simulink model "ModeloOpal"  (R2017a)
settings: Solver=ode4  StartTime=0.0  StopTime=inf  FixedStep=Ts  RelTol=1e-3  EnableMultiTasking=on
PostLoadFcn:
  | Ts=1/100080;L=1.8e-3;w=2*pi*60;C=20e-6;
  | 
  | load('CycleFTP75.mat')
  | 
  | Vel=Cycle(:,1);
  | Acc=Cycle(:,2);
InitFcn:
  | Ts=1/100080;L=1.8e-3;w=2*pi*60;C=20e-6;
  | 
  | load('CycleFTP75.mat')
  | 
  | Vel=Cycle(:,1);
  | Acc=Cycle(:,2);
undefined symbols (not defined in the file): DiscIntNeverNeededParam, OP4510_1B_Ch00, OP4510_2A_Ch00, OP4510_2A_Ch08, OP4510_2B_Ch00, OP4510_2B_Ch08, sizecont
libraries: rtlab x29, simulink x5, dspswit3 x2
(part 1 of 2)
Description:
  | Model of a simple control system for use iin training.
settings Model: Creator=Paul Baracos  LastModifiedBy=LIFAE
settings SolverCC: InsertRTBMode=Never (minimum delay)
settings DataIOCC: LimitDataPoints=on  SaveFormat=Array  SaveOutput=off  SaveTime=off  SignalLoggingName=sigsOut
settings OptimizationCC: BlockReduction=off  BooleanDataType=off  OptimizeBlockIOStorage=off  BufferReuse=off  GlobalBufferReuse=off  ExpressionFolding=off  LocalBlockOutputs=off  InitFltsAndDblsToZero=on  LifeSpan=inf
settings DebuggingCC: SaveWithParameterizedLinksMsg=none  UnderspecifiedInitializationDetection=Classic  MergeDetectMultiDrivingBlocksExec=none  SignalResolutionControl=TryResolveAllWithWarning  MultiTaskDSMMsg=warning  MultiTaskCondExecSysMsg=none  FcnCallInpInsideContextMsg=warning  SFUnexpectedBacktrackingDiag=warning  SFNoUnconditionalDefaultTransitionDiag=warning  SFExecutionAtInitializationDiag=none
settings HardwareCC: ProdBitPerPointer=32  ProdBitPerSizeT=32  ProdBitPerPtrDiffT=32  ProdLargestAtomicFloat=None  ProdIntDivRoundTo=Undefined  ProdEndianess=Unspecified  ProdWordSize=32  ProdHWDeviceType=32-bit Generic  TargetBitPerPointer=64  TargetBitPerSizeT=64  TargetBitPerPtrDiffT=64  TargetLongLongMode=on  TargetIntDivRoundTo=Zero  TargetEndianess=LittleEndian  TargetWordSize=64  TargetHWDeviceType=MATLAB Host  ProdEqTarget=off
settings ModelReferenceCC: PropagateSignalLabelsOutOfModel=off
settings GRTTargetCC: TargetFcnLib=ansi_tfl_tmw.mat  TargetLangStandard=C89/C90 (ANSI)  CombineOutputUpdateFcns=off  GRTInterface=on
settings ConfigComp: CovMetricSettings=dw  CovSaveCumulativeToWorkspaceVar=on  CovSaveSingleToWorkspaceVar=on  CovExternalEMLEnable=off

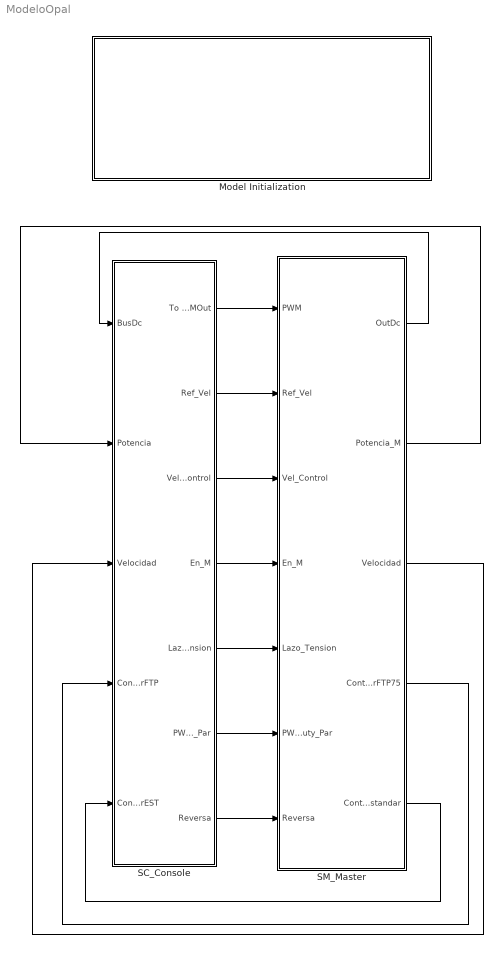
== system ModeloOpal ==
  Model Initialization : Subsystem  AncestorBlock=artemis/Tools /Misc/Model Initialization  mask(Model Functions){InitFcnX=|, prel=off, posl=on, inif=on, strf=off}
      mask InitFcnX=|
      | Ts=1/100080;L=1.8e-3;w=2*pi*60;C=20e-6;
      |
      | load('CycleFTP75.mat')
      |
      | Vel=Cycle(:,1);
      | Acc=Cycle(:,2);
      mask prompts: InitFcnX "Initialisation"; prel "Preload Function"; posl "PostLoad Function"; inif "InitFcn"; strf "StartFcn"
      mask init:
      | currentBlock = gcb;
      | root = bdroot(currentBlock);
      | 
      | if ~strcmp(get_param(root,'BlockDiagramType'),'library')
      |     if prel==1
      |         set_param(root, 'PreLoadFcn', InitFcnX);
      |     else
      |         set_param(root, 'PreLoadFcn', '');
      |     end
      |     if inif==1
      |         set_param(root, 'InitFcn', InitFcnX);
      |     else
      |         set_param(root, 'InitFcn', '');
      |     end
      |     if strf==1
      |         set_param(root, 'StartFcn', InitFcnX);
      |     else
      |         set_param(root, 'StartFcn', '');
      |     end
      |     if posl==1
      |         set_param(root, 'PostLoadFcn', InitFcnX);
      |     else
      |         set_param(root, 'PostLoadFcn', '');
      |     end
      | end
      | 
      | pos = get_param(currentBlock, 'Position');
      | width = pos(3) - pos(1); height = pos(4) - pos(2);
      | txt = [ upper(root) '\n' '- InitFcn. . . . . '  get_param(root, 'InitFcn') ];
      settings: CopyFcn=set_param(gcb,'LinkStatus','inactive')
      mask Display: text(5, height*0.5, txt, 'horizontalAlignment', 'left', 'verticalAlignment', 'middle') ;
  SC_Console : Subsystem
  SM_Master : Subsystem
  wires:
  SM_Master/1("OutDc ") -> SC_Console/1(BusDc)
  SM_Master/2(Potencia_M) -> SC_Console/2(Potencia)
  SC_Console/1(To PWMOut) -> SM_Master/1("PWM ")
  SM_Master/3(Velocidad) -> SC_Console/3(Velocidad)
  SM_Master/4(ContadorFTP75) -> SC_Console/4(ContadorFTP)
  SM_Master/5(ContadorEstandar) -> SC_Console/5(ContadorEST)
  SC_Console/2(Ref_Vel) -> SM_Master/2(Ref_Vel)
  SC_Console/3(Vel_Control) -> SM_Master/3(Vel_Control)
  SC_Console/4(En_M) -> SM_Master/4(En_M)
  SC_Console/5("Lazo_Tension ") -> SM_Master/5(Lazo_Tension)
  SC_Console/6(PWM_Duty_Par) -> SM_Master/6(PWM_Duty_Par)
  SC_Console/7(Reversa) -> SM_Master/7(Reversa)

== system ModeloOpal/Model Initialization ==

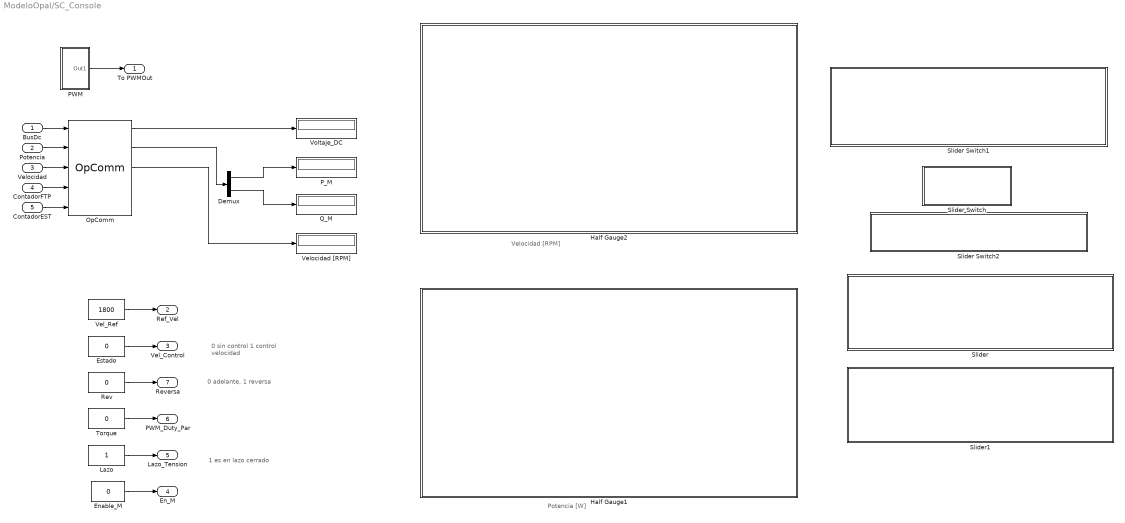
== system ModeloOpal/SC_Console ==
  note: Velocidad [RPM]
  note: 0 sin control
      | 1 control velocidad
  note: 0 adelante, 1 reversa
  note: 1 es en lazo cerrado
  note: Potencia [W]
  BusDc : Inport
  Potencia : Inport  Port=2
  Velocidad : Inport  Port=3
  ContadorFTP : Inport  Port=4
  ContadorEST : Inport  Port=5
  Demux : Demux  Outputs=2
  Enable_M : Constant  Value=0
  Estado : Constant  Value=0
  Half Gauge1 : Subsystem  DialogController=hmiCreateDDGDialog  IsWebBlock=on  mask(MWDashboardBlock){webBlockId=9bf2f812-ab57-4af6-888e-ff456dd2f0e9, webBlockType=semicirculargauge, ShowInLibBrowser=on, ShowInitialText=on, HMISrcModelName=EV}
      mask prompts: webBlockId "WebBlock Id"; webBlockType "WebBlock Type"; HMISrcModelName "Source Model"
      mask help: SimulinkHMI:dialogs:SemicircularGaugeDialogDesc
      mask Help: helpview([docroot '/mapfiles/simulink.map'], 'hmi_half_gauge')
      mask Display:
      | if strcmp(get_param(bdroot(gcb),'BlockDiagramType'), 'library')
      |     image([(matlabroot) '/toolbox/simulink/hmi/icons/SemicircularGauge.png']);
      | end
  Half Gauge2 : Subsystem  DialogController=hmiCreateDDGDialog  IsWebBlock=on  mask(MWDashboardBlock){webBlockId=4c0e6855-45c1-4807-b490-75edbe862d8f, webBlockType=semicirculargauge, ShowInLibBrowser=on, ShowInitialText=on, HMISrcModelName=EV}
      mask prompts: webBlockId "WebBlock Id"; webBlockType "WebBlock Type"; HMISrcModelName "Source Model"
      mask help: SimulinkHMI:dialogs:SemicircularGaugeDialogDesc
      mask Help: helpview([docroot '/mapfiles/simulink.map'], 'hmi_half_gauge')
      mask Display:
      | if strcmp(get_param(bdroot(gcb),'BlockDiagramType'), 'library')
      |     image([(matlabroot) '/toolbox/simulink/hmi/icons/SemicircularGauge.png']);
      | end
  Lazo : Constant
  OpComm : rtlab/OpComm  nbport=5  groupe_acq=1  subsys_rate=0  st=0  Synchronization=on  Interpolation=on  Threshold=1.0  Missed_Data=off  Sim_Time=off  Samples=off  dynSigOut=off  from_console=0  warning_done=off  writeOpCommFile=off  Offset=off
      settings: SourceProductName=RT-LAB
  PWM : Subsystem
  P_M : Display
  Q_M : Display
  Rev : Constant  Value=0
  Slider : Subsystem  DialogController=hmiCreateDDGDialog  IsWebBlock=on  mask(MWDashboardBlock){webBlockId=662892dd-7b3a-463b-8f2b-6a3bb7b3c375, webBlockType=slider, ShowInLibBrowser=on, ShowInitialText=on, HMISrcModelName=EV}
      mask prompts: webBlockId "WebBlock Id"; webBlockType "WebBlock Type"; HMISrcModelName "Source Model"
      mask help: SimulinkHMI:dialogs:SliderDialogDesc
      mask Help: helpview([docroot '/mapfiles/simulink.map'], 'hmi_slider')
      mask Display:
      | if strcmp(get_param(bdroot(gcb),'BlockDiagramType'), 'library')
      |     image([(matlabroot) '/toolbox/simulink/hmi/icons/Slider.png']);
      | end
  Slider Switch : Subsystem  DialogController=hmiCreateDDGDialog  IsWebBlock=on  mask(MWDashboardBlock){webBlockId=e4e01401-8b8e-4eb0-8cfa-0b1290c49f07, webBlockType=sliderswitch, ShowInLibBrowser=on, ShowInitialText=on, HMISrcModelName=EV}
      mask prompts: webBlockId "WebBlock Id"; webBlockType "WebBlock Type"; HMISrcModelName "Source Model"
      mask help: SimulinkHMI:dialogs:SwitchDialogDesc
      mask Help: helpview([docroot '/mapfiles/simulink.map'], 'hmi_slider_switch')
      mask Display:
      | if strcmp(get_param(bdroot(gcb),'BlockDiagramType'), 'library')
      |     image([(matlabroot) '/toolbox/simulink/hmi/icons/SliderSwitch.png']);
      | end
  Slider Switch1 : Subsystem  DialogController=hmiCreateDDGDialog  IsWebBlock=on  mask(MWDashboardBlock){webBlockId=fdde9750-0d4e-4e96-acc9-80e84340a54d, webBlockType=sliderswitch, ShowInLibBrowser=on, ShowInitialText=on, HMISrcModelName=EV}
      mask prompts: webBlockId "WebBlock Id"; webBlockType "WebBlock Type"; HMISrcModelName "Source Model"
      mask help: SimulinkHMI:dialogs:SwitchDialogDesc
      mask Help: helpview([docroot '/mapfiles/simulink.map'], 'hmi_slider_switch')
      mask Display:
      | if strcmp(get_param(bdroot(gcb),'BlockDiagramType'), 'library')
      |     image([(matlabroot) '/toolbox/simulink/hmi/icons/SliderSwitch.png']);
      | end
  Slider Switch2 : Subsystem  DialogController=hmiCreateDDGDialog  IsWebBlock=on  mask(MWDashboardBlock){webBlockId=cc9abc73-cb6f-40c5-b477-d0f2468ee603, webBlockType=sliderswitch, ShowInLibBrowser=on, ShowInitialText=on, HMISrcModelName=EV}
      mask prompts: webBlockId "WebBlock Id"; webBlockType "WebBlock Type"; HMISrcModelName "Source Model"
      mask help: SimulinkHMI:dialogs:SwitchDialogDesc
      mask Help: helpview([docroot '/mapfiles/simulink.map'], 'hmi_slider_switch')
      mask Display:
      | if strcmp(get_param(bdroot(gcb),'BlockDiagramType'), 'library')
      |     image([(matlabroot) '/toolbox/simulink/hmi/icons/SliderSwitch.png']);
      | end
  Slider1 : Subsystem  DialogController=hmiCreateDDGDialog  IsWebBlock=on  mask(MWDashboardBlock){webBlockId=d9866bfa-8e08-4068-9fd6-1c09dd8bbfc2, webBlockType=slider, ShowInLibBrowser=on, ShowInitialText=on, HMISrcModelName=EV}
      mask prompts: webBlockId "WebBlock Id"; webBlockType "WebBlock Type"; HMISrcModelName "Source Model"
      mask help: SimulinkHMI:dialogs:SliderDialogDesc
      mask Help: helpview([docroot '/mapfiles/simulink.map'], 'hmi_slider')
      mask Display:
      | if strcmp(get_param(bdroot(gcb),'BlockDiagramType'), 'library')
      |     image([(matlabroot) '/toolbox/simulink/hmi/icons/Slider.png']);
      | end
  Torque : Constant  Value=0
  Vel_Ref : Constant  Value=1800
  Velocidad [RPM] : Display
  Voltaje_DC : Display
  To PWMOut : Outport
  Ref_Vel : Outport  Port=2
  Vel_Control : Outport  Port=3
  En_M : Outport  Port=4
  "Lazo_Tension " : Outport  Port=5
  PWM_Duty_Par : Outport  Port=6
  Reversa : Outport  Port=7
  wires:
  BusDc/1 -> OpComm/1
  OpComm/1 -> Voltaje_DC/1
  Potencia/1 -> OpComm/2
  OpComm/2 -> Demux/1
  Demux/1 -> P_M/1
  Demux/2 -> Q_M/1
  PWM/1(Out1) -> To PWMOut/1
  Enable_M/1 -> En_M/1
  Lazo/1 -> "Lazo_Tension "/1
  Torque/1 -> PWM_Duty_Par/1
  Velocidad/1 -> OpComm/3
  OpComm/3 -> Velocidad [RPM]/1
  ContadorFTP/1 -> OpComm/4
  Rev/1 -> Reversa/1
  Estado/1 -> Vel_Control/1
  Vel_Ref/1 -> Ref_Vel/1
  ContadorEST/1 -> OpComm/5

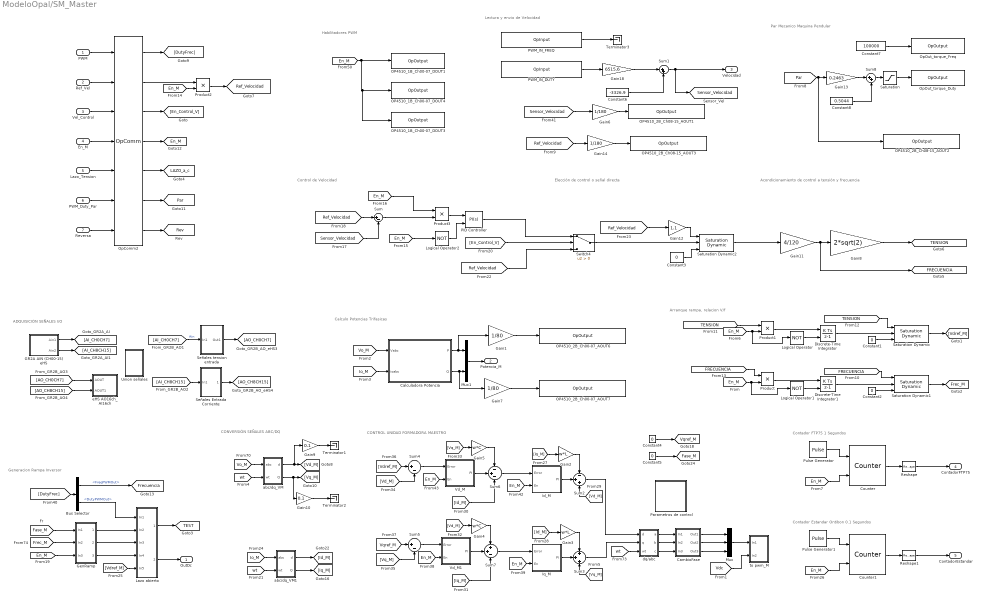
== system ModeloOpal/SM_Master ==
  note: Lectura y envio de Velocidad
  note: Calculo Potencias Trifasicas
  note: Generacion Rampa Inversor
  note: Arranque rampa, relacion V/f
  note: Par Mecanico Maquina Pendular
  note: Contador FTP75 1 Segundos
  note: Acondicionamiento de control a tensión y frecuencia
  note: Elección de control o señal directa
  note: Control de Velocidad
  note: Habilitadores PWM
  note: ADQUISICIÓN SEÑALES I/O
  note: CONVERSIÓN SEÑALES ABC/DQ
  note: CONTROL UNIDAD FORMADORA MAESTRO
  note: Contador Estandar Ontibon 0.1 Segundos
  "PWM " : Inport
  Ref_Vel : Inport  Port=2
  Vel_Control : Inport  Port=3
  En_M : Inport  Port=4
  Lazo_Tension : Inport  Port=5
  PWM_Duty_Par : Inport  Port=6
  Reversa : Inport  Port=7
  Bus Selector : BusSelector  OutputSignals=FreqPWMOut,DutyPWMOut
  Calculadora Potencia : Subsystem
  CambioFase : Subsystem
  Constant{1..5} (5 alike) : Constant  Value=0
  Constant6 : Constant  Value=-3326.9
  Constant7 : Constant  Value=100000
  Constant8 : Constant  Value=0.5044
  Counter : dspswit3/Counter  Direction=Up  CountEvent=Rising edge  CounterSize=User defined  MaxCount=2474  InitialCount=0  Output=Count  HitValue=sizecont-1  ResetInput=on  SamplesPerFrame=1  Ts=1  CntDtype=double  HitDtype=Logical
  Counter1 : dspswit3/Counter  Direction=Up  CountEvent=Rising edge  CounterSize=User defined  MaxCount=2474  InitialCount=0  Output=Count  HitValue=sizecont-1  ResetInput=on  SamplesPerFrame=1  Ts=1  CntDtype=double  HitDtype=Logical
  Discrete-Time Integrator : DiscreteIntegrator  ExternalReset=level  InitialConditionSetting=State (most efficient)  SampleTime=-1  ICPrevOutput=DiscIntNeverNeededParam  ICPrevScaledInput=DiscIntNeverNeededParam
  Discrete-Time Integrator1 : DiscreteIntegrator  ExternalReset=level  InitialConditionSetting=State (most efficient)  SampleTime=-1  ICPrevOutput=DiscIntNeverNeededParam  ICPrevScaledInput=DiscIntNeverNeededParam
  GR2A AIN (CH00-15) eHS : Subsystem
  Gain1 : Gain  Gain=1/80
  Gain10 : Gain  Gain=0.1
  Gain11 : Gain  Gain=4/120
  Gain12 : Gain  Gain=1.1
  Gain13 : Gain  Gain=0.2463
  Gain14 : Gain  Gain=1/180
  Gain18 : Gain  Gain=6515.6
  Gain2 : Gain  Gain=w*L
  Gain3 : Gain  Gain=w*L
  Gain4 : Gain  Gain=w*C
  Gain5 : Gain  Gain=w*C
  Gain6 : Gain  Gain=1/180
  Gain7 : Gain  Gain=1/80
  Gain8 : Gain  Gain=2*sqrt(2)  SaturateOnIntegerOverflow=on  OutDataTypeStr=Inherit: Same as input  ParamDataTypeStr=Inherit: Same as input
  Gain9 : Gain  Gain=0.1
  GenRamp : Subsystem
  Id_M : Subsystem
  Iq_M : Subsystem
  "Lazo abierto " : Subsystem
  Logical Operator : Logic  Operator=NOT  AllPortsSameDT=off  OutDataTypeStr=boolean
  Logical Operator1 : Logic  Operator=NOT  AllPortsSameDT=off  OutDataTypeStr=boolean
  Logical Operator2 : Logic  Operator=NOT  AllPortsSameDT=off  OutDataTypeStr=boolean
  Mux : Mux  Inputs=3
  Mux1 : Mux  Inputs=2
  OP4510_1B_Ch00-07_DOUT1 : rtlab/OpOutput  identifier_use=[]  identifier_hide=OP4510_1B_Ch00-07_DOUT1  nb_parents_identifier=0
      settings: SourceProductName=RT-LAB
  OP4510_1B_Ch00-07_DOUT3 : rtlab/OpOutput  identifier_use=[]  identifier_hide=OP4510_1B_Ch00-07_DOUT3  nb_parents_identifier=0
      settings: SourceProductName=RT-LAB
  OP4510_1B_Ch00-07_DOUT4 : rtlab/OpOutput  identifier_use=[]  identifier_hide=OP4510_1B_Ch00-07_DOUT4  nb_parents_identifier=0
      settings: SourceProductName=RT-LAB
  OP4510_2B_Ch00-07_AOUT6 : rtlab/OpOutput  identifier_use=[]  identifier_hide=OP4510_2B_Ch00-07_AOUT6  nb_parents_identifier=0
      settings: SourceProductName=RT-LAB
  OP4510_2B_Ch00-07_AOUT7 : rtlab/OpOutput  identifier_use=[]  identifier_hide=OP4510_2B_Ch00-07_AOUT7  nb_parents_identifier=0
      settings: SourceProductName=RT-LAB
  OP4510_2B_Ch08-15_AOUT1 : rtlab/OpOutput  identifier_use=[]  identifier_hide=OP4510_2B_Ch08-15_AOUT1  nb_parents_identifier=0
      settings: SourceProductName=RT-LAB
  OP4510_2B_Ch08-15_AOUT2 : rtlab/OpOutput  identifier_use=[]  identifier_hide=OP4510_2B_Ch08-15_AOUT2  nb_parents_identifier=0
      settings: SourceProductName=RT-LAB
  OP4510_2B_Ch08-15_AOUT3 : rtlab/OpOutput  identifier_use=[]  identifier_hide=OP4510_2B_Ch08-15_AOUT3  nb_parents_identifier=0
      settings: SourceProductName=RT-LAB
  OpComm2 : rtlab/OpComm  nbport=7  groupe_acq=1  subsys_rate=0  st=0  Synchronization=on  Interpolation=on  Threshold=1.0  Missed_Data=off  Sim_Time=off  Samples=off  dynSigOut=off  from_console=1  warning_done=off  writeOpCommFile=off  Offset=off
      settings: SourceProductName=RT-LAB
  OpOut_torque_Duty : rtlab/OpOutput  identifier_use=[]  identifier_hide=OpOut_torque_Duty  nb_parents_identifier=0
      settings: SourceProductName=RT-LAB
  OpOut_torque_Freq : rtlab/OpOutput  identifier_use=[]  identifier_hide=OpOut_torque_Freq  nb_parents_identifier=0
      settings: SourceProductName=RT-LAB
  PID Controller : simulink/Continuous/PID Controller  Controller=PI  TimeDomain=Continuous-time  SampleTime=-1  IntegratorMethod=Forward Euler  FilterMethod=Forward Euler  Form=Parallel  UseFilter=on  ControllerParametersSource=internal  P=0.502  I=21.7  D=0  N=100  InitialConditionSource=internal  InitialConditionForIntegrator=0  InitialConditionForFilter=0  ExternalReset=level  LimitOutput=off  UpperSaturationLimit=inf  LowerSaturationLimit=-inf  LinearizeAsGain=on  AntiWindupMode=none  Kb=1  TrackingMode=off  Kt=1  PParamMin=[]  PParamMax=[]  IParamMin=[]  IParamMax=[]  DParamMin=[]  DParamMax=[]  NParamMin=[]  NParamMax=[]  KbParamMin=[]  KbParamMax=[]  KtParamMin=[]  KtParamMax=[]  POutMin=[]  POutMax=[]  IOutMin=[]  IOutMax=[]  DOutMin=[]  DOutMax=[]  NOutMin=[]  NOutMax=[]  KbOutMin=[]  KbOutMax=[]  KtOutMin=[]  KtOutMax=[]  IntegratorOutMin=[]  IntegratorOutMax=[]  FilterOutMin=[]  FilterOutMax=[]  SumOutMin=[]  SumOutMax=[]  SumI1OutMin=[]  SumI1OutMax=[]  SumI2OutMin=[]  SumI2OutMax=[]  SumI3OutMin=[]  SumI3OutMax=[]  SumDOutMin=[]  SumDOutMax=[]  SaturationOutMin=[]  SaturationOutMax=[]  IntegratorContinuousStateAttributes=''  IntegratorStateMustResolveToSignalObject=off  IntegratorRTWStateStorageClass=Auto  FilterContinuousStateAttributes=''  FilterStateMustResolveToSignalObject=off  FilterRTWStateStorageClass=Auto  DifferentiatorICPrevScaledInput=0  DifferentiatorOutMin=[]  DifferentiatorOutMax=[]  InitialConditionSetting=State (most efficient)
  PWM_IN_DUTY : rtlab/OpInput  identifier_use=[]  identifier_hide=PWM_IN_DUTY  nb_parents_identifier=0  passthrough=off  init_value=0  value_type=double  create_alias=on
      settings: SourceProductName=RT-LAB
  PWM_IN_FREQ : rtlab/OpInput  identifier_use=[]  identifier_hide=PWM_IN_FREQ  nb_parents_identifier=0  passthrough=off  init_value=0  value_type=double  create_alias=on
      settings: SourceProductName=RT-LAB
  Parametros de control : Subsystem
  Product{,1..3} (4 alike) : Product
  Pulse Generator : DiscretePulseGenerator  PulseType=Time based  Period=1  PulseWidth=5
  Pulse Generator1 : DiscretePulseGenerator  PulseType=Time based  Period=1  PulseWidth=5
  Reshape : Reshape  OutputDimensionality=Customize  OutputDimensions=[1]
  Reshape1 : Reshape  OutputDimensionality=Customize  OutputDimensions=[1]
  Saturation : Saturate  UpperLimit=1  LowerLimit=0
  Saturation Dynamic : simulink/Discontinuities/Saturation Dynamic  OutMin=[]  OutMax=[]  OutDataTypeStr=Inherit: Same as second input  OutDataType=fixdt(1, 16)  OutScaling=2^-10  DoSatur=off
  Saturation Dynamic1 : simulink/Discontinuities/Saturation Dynamic  OutMin=[]  OutMax=[]  OutDataTypeStr=Inherit: Same as second input  OutDataType=fixdt(1, 16)  OutScaling=2^-10  DoSatur=off
  Saturation Dynamic2 : simulink/Discontinuities/Saturation Dynamic  OutMin=[]  OutMax=[]  OutDataTypeStr=Inherit: Same as second input  OutDataType=fixdt(1, 16)  OutScaling=2^-10  DoSatur=off
  Señales Entrada Corriente : Subsystem
  Señales tension entrada : Subsystem
  Sum : Sum  Inputs=|+-
  Sum1 : Sum  Inputs=|++
  Sum2 : Sum  Inputs=-++
  Sum3 : Sum  Inputs=+++
  Sum4 : Sum  Inputs=|+-
  Sum5 : Sum  Inputs=|+-
  Sum6 : Sum  Inputs=-+-
  Sum7 : Sum  Inputs=++-
  Sum8 : Sum  Inputs=|++
  Switch4 : Switch  Criteria=u2 > Threshold
  Terminator1 : Terminator
  Terminator2 : Terminator
  Terminator3 : Terminator
  "Union señales " : Subsystem
  Vd_M : Subsystem
  Vd_M1 : Subsystem
  abc/dq_VM : Subsystem
  abc/dq_VM1 : Subsystem
  dq/abc : Subsystem
  eHS AO16ch_AI16ch : Subsystem
  to pwm_M : Subsystem
  "OutDc " : Outport
  Potencia_M : Outport  Port=2
  Velocidad : Outport  Port=3
  ContadorFTP75 : Outport  Port=4
  ContadorEstandar : Outport  Port=5
  tag scope: En_M=global, FRECUENCIA=global, Fase_M=global, Frec_M=global, Frecuencia=global, LAZO_a_c=global, Par=global, Ref_Velocidad=global, Rev=global, Sensor_Velocidad=global, TENSION=global, TEST=global, Vqref_M=global
  wires:
  [Frec_M] -> GenRamp/2(In2)
  [En_M] -> GenRamp/3(In3)
  [Fase_M] -> GenRamp/1(In1)
  [AO_CH0CH7] -> eHS AO16ch_AI16ch/1(AOUT)
  [AO_CH8CH15] -> eHS AO16ch_AI16ch/2(AOUT1)
  GR2A AIN (CH00-15) eHS/1(Ain1) -> [AI_CH0CH7]
  GR2A AIN (CH00-15) eHS/2(Ain2) -> [AI_CH8CH15]
  [AI_CH0CH7] -> Señales tension entrada/1(In1)  "Ain"
  Señales tension entrada/1(Out1) -> [AO_CH0CH7]
  [AI_CH8CH15] -> Señales Entrada Corriente/1(In1)
  Señales Entrada Corriente/1(Out1) -> [AO_CH8CH15]
  GenRamp/1(Out1) -> "Lazo abierto "/2(In2)
  GenRamp/2(Out2) -> "Lazo abierto "/3(In3)
  GenRamp/3(Out3) -> "Lazo abierto "/4(In4)
  "Lazo abierto "/2(Out2) -> "OutDc "/1
  "Lazo abierto "/1(Out1) -> [TEST]
  [Vo_M] -> Calculadora Potencia/1(Vabc)
  [Io_M] -> Calculadora Potencia/2(ioabc)
  Calculadora Potencia/2("Q ") -> Gain7/1, Mux1/2
  Calculadora Potencia/1(P) -> Gain1/1, Mux1/1
  Mux1/1 -> Potencia_M/1
  [En_M] -> OP4510_1B_Ch00-07_DOUT1/1, OP4510_1B_Ch00-07_DOUT4/1, OP4510_1B_Ch00-07_DOUT3/1
  "PWM "/1 -> OpComm2/1
  Bus Selector/1 -> [Frecuencia]  "<FreqPWMOut>"
  [En_M] -> Logical Operator1/1, Product/2
  Product/1 -> Discrete-Time Integrator1/1
  Product1/1 -> Discrete-Time Integrator/1
  [En_M] -> Logical Operator/1, Product1/2
  Logical Operator/1 -> Discrete-Time Integrator/2
  Logical Operator1/1 -> Discrete-Time Integrator1/2
  Discrete-Time Integrator/1 -> Saturation Dynamic/2
  Saturation Dynamic/1 -> [Vdref_M]
  Discrete-Time Integrator1/1 -> Saturation Dynamic1/2
  Saturation Dynamic1/1 -> [Frec_M]
  Bus Selector/2 -> "Lazo abierto "/1(In1)  "<DutyPWMOut>"
  [Vdref_M] -> Sum4/1
  Id_M/1(PI) -> Sum2/2
  [Vo_M] -> abc/dq_VM/1(abc)
  Gain9/1 -> Terminator1/1
  [Vdc] -> to pwm_M/2(In2)
  abc/dq_VM/1(d) -> Gain9/1, [Vd_M]
  [En_M] -> Vd_M/2(En)
  [En_M] -> Id_M/2(En)
  [wt] -> abc/dq_VM/2(wt)
  Vd_M1/1(PI) -> Sum7/2
  [Vd_M] -> Sum4/2
  [En_M] -> Iq_M/2(En)
  Sum7/1 -> Iq_M/1(Error)
  Mux/1 -> to pwm_M/1(In1)
  Sum4/1 -> Vd_M/1(Error)
  Iq_M/1(PI) -> Sum3/2
  [Iq_M] -> Gain2/1
  Gain4/1 -> Sum7/1
  Sum3/1 -> dq/abc/2(q)
  [Vd_M] -> Gain4/1
  Vd_M/1(PI) -> Sum6/2
  [En_M] -> Vd_M1/2(En)
  abc/dq_VM1/1(d) -> [Id_M]
  [wt] -> dq/abc/3(wt)
  [Id_M] -> Gain3/1
  [Vq_M] -> Sum3/3
  [Vq_M] -> Gain5/1
  [Vq_M] -> Sum5/2
  Sum2/1 -> dq/abc/1(d)
  Gain5/1 -> Sum6/1
  [Vqref_M] -> Sum5/1
  Gain2/1 -> Sum2/1
  Sum6/1 -> Id_M/1(Error)
  [Id_M] -> Sum6/3
  [Iq_M] -> Sum7/3
  [Vd_M] -> Sum2/3
  Gain3/1 -> Sum3/1
  abc/dq_VM1/2(Q) -> [Iq_M]
  Gain10/1 -> Terminator2/1
  [Io_M] -> abc/dq_VM1/1(abc)
  abc/dq_VM/2(Q) -> Gain10/1, [Vq_M]
  [wt] -> abc/dq_VM1/2(wt)
  Sum5/1 -> Vd_M1/1(Error)
  PWM_IN_FREQ/1 -> Terminator3/1
  Constant2/1 -> Saturation Dynamic1/3
  Pulse Generator/1 -> Counter/1
  [En_M] -> Counter/2
  Reshape/1 -> ContadorFTP75/1
  Counter/1 -> Reshape/1
  Gain1/1 -> OP4510_2B_Ch00-07_AOUT6/1
  Gain7/1 -> OP4510_2B_Ch00-07_AOUT7/1
  Constant6/1 -> Sum1/2
  Gain18/1 -> Sum1/1
  Sum1/1 -> [Sensor_Velocidad], Velocidad/1
  PWM_IN_DUTY/1 -> Gain18/1
  Gain11/1 -> Gain8/1, [FRECUENCIA]
  Gain8/1 -> [TENSION]
  [TENSION] -> Product1/1
  [TENSION] -> Saturation Dynamic/1
  [FRECUENCIA] -> Saturation Dynamic1/1
  [FRECUENCIA] -> Product/1
  Constant3/1 -> Saturation Dynamic2/3
  Saturation Dynamic2/1 -> Gain11/1
  Gain12/1 -> Saturation Dynamic2/1
  [En_M] -> Logical Operator2/1
  Logical Operator2/1 -> PID Controller/2
  Product3/1 -> PID Controller/1
  Sum/1 -> Product3/2
  [En_M] -> Product3/1
  PID Controller/1 -> Switch4/1
  [Sensor_Velocidad] -> Sum/2
  [En_M] -> Product2/2
  Product2/1 -> [Ref_Velocidad]
  [Ref_Velocidad] -> Sum/1
  [En_Control_V] -> Switch4/2
  [Ref_Velocidad] -> Switch4/3
  Switch4/1 -> Saturation Dynamic2/2
  [Ref_Velocidad] -> Gain12/1
  Constant1/1 -> Saturation Dynamic/3
  [Vdref_M] -> "Lazo abierto "/5(In5)
  Constant4/1 -> [Vqref_M]
  Constant5/1 -> [Fase_M]
  Counter1/1 -> Reshape1/1
  Pulse Generator1/1 -> Counter1/1
  Reshape1/1 -> ContadorEstandar/1
  [En_M] -> Counter1/2
  Ref_Vel/1 -> OpComm2/2
  Vel_Control/1 -> OpComm2/3
  OpComm2/2 -> Product2/1
  En_M/1 -> OpComm2/4
  Lazo_Tension/1 -> OpComm2/5
  OpComm2/4 -> [En_M]
  OpComm2/5 -> [LAZO_a_c]
  OpComm2/3 -> [En_Control_V]
  OpComm2/1 -> [DutyFrec]
  [DutyFrec] -> Bus Selector/1
  dq/abc/1(a) -> CambioFase/1(In1)
  dq/abc/2(b) -> CambioFase/2(In2)
  dq/abc/3(c) -> CambioFase/3(In3)
  CambioFase/1(Out1) -> Mux/1
  CambioFase/2(Out2) -> Mux/2
  CambioFase/3(Out3) -> Mux/3
  Constant7/1 -> OpOut_torque_Freq/1
  PWM_Duty_Par/1 -> OpComm2/6
  Reversa/1 -> OpComm2/7
  OpComm2/7 -> [Rev]
  OpComm2/6 -> [Par]
  Gain13/1 -> Sum8/1
  Constant8/1 -> Sum8/2
  [Par] -> OP4510_2B_Ch08-15_AOUT2/1, Gain13/1
  Sum8/1 -> Saturation/1
  Saturation/1 -> OpOut_torque_Duty/1
  [Ref_Velocidad] -> Gain14/1
  Gain14/1 -> OP4510_2B_Ch08-15_AOUT3/1
  Gain6/1 -> OP4510_2B_Ch08-15_AOUT1/1
  [Sensor_Velocidad] -> Gain6/1

== system ModeloOpal/SC_Console/Half Gauge1 ==

== system ModeloOpal/SC_Console/Half Gauge2 ==

== system ModeloOpal/SC_Console/PWM ==
  A1 : Constant  Value=20
  B1 : Constant  Value=10080
  Bus Creator : BusCreator  Inputs=3
  Bus Creator2 : BusCreator  Inputs=3
  Bus Creator3 : BusCreator  Inputs=2
  Out1 : Outport
  wires:
  Bus Creator2/1 -> Bus Creator3/1  "FreqPWMOut"
  Bus Creator/1 -> Bus Creator3/2  "DutyPWMOut"
  Bus Creator3/1 -> Out1/1  "PWMO_Ch00_07"
  A1/1 -> Bus Creator/2, Bus Creator/3, Bus Creator/1  "DutyCh02"
  B1/1 -> Bus Creator2/1, Bus Creator2/2, Bus Creator2/3  "FreqCh00"

== system ModeloOpal/SC_Console/Slider ==

== system ModeloOpal/SC_Console/Slider Switch ==

== system ModeloOpal/SC_Console/Slider Switch1 ==

== system ModeloOpal/SC_Console/Slider Switch2 ==

== system ModeloOpal/SC_Console/Slider1 ==

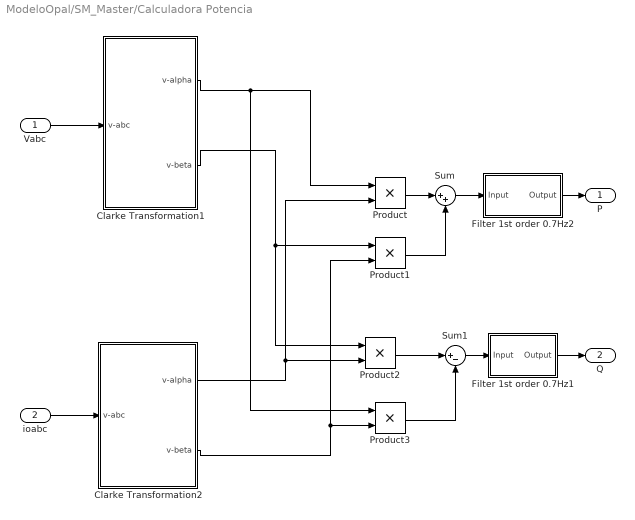
== system ModeloOpal/SM_Master/Calculadora Potencia ==
  Vabc : Inport
  ioabc : Inport  Port=2
  Clarke Transformation1 : Subsystem
  Clarke Transformation2 : Subsystem
  Filter 1st order 0.7Hz1 : Subsystem  Tag=FilterWizardSubSystem
      settings: ErrorFcn=dspFilterRealizedInBasicElemsAlgLoopErrFcnCallback
  Filter 1st order 0.7Hz2 : Subsystem  Tag=FilterWizardSubSystem
      settings: ErrorFcn=dspFilterRealizedInBasicElemsAlgLoopErrFcnCallback
  Product{,1..3} (4 alike) : Product  RndMeth=Zero
  Sum : Sum  Inputs=|++
  Sum1 : Sum  Inputs=|+-
  P : Outport
  "Q " : Outport  Port=2
  wires:
  Vabc/1 -> Clarke Transformation1/1(v-abc)
  ioabc/1 -> Clarke Transformation2/1(v-abc)
  Product/1 -> Sum/1
  Product1/1 -> Sum/2
  Product2/1 -> Sum1/1
  Product3/1 -> Sum1/2
  Sum/1 -> Filter 1st order 0.7Hz2/1(Input)
  Sum1/1 -> Filter 1st order 0.7Hz1/1(Input)
  Clarke Transformation1/1(v-alpha) -> Product3/1, Product/1
  Clarke Transformation1/2(v-beta) -> Product1/1, Product2/1
  Clarke Transformation2/1(v-alpha) -> Product2/2, Product/2
  Clarke Transformation2/2(v-beta) -> Product3/2, Product1/2
  Filter 1st order 0.7Hz1/1(Output) -> "Q "/1
  Filter 1st order 0.7Hz2/1(Output) -> P/1

== system ModeloOpal/SM_Master/CambioFase ==
  In1 : Inport
  In2 : Inport  Port=2
  In3 : Inport  Port=3
  Switch1 : Switch  Criteria=u2 > Threshold
  Switch2 : Switch  Criteria=u2 > Threshold
  Out1 : Outport
  Out2 : Outport  Port=2
  Out3 : Outport  Port=3
  wires:
  Switch1/1 -> Out1/1
  [Rev] -> Switch2/2
  [Rev] -> Switch1/2
  In1/1 -> Switch2/1, Switch1/3
  In2/1 -> Out2/1
  In3/1 -> Switch2/3, Switch1/1
  Switch2/1 -> Out3/1

== system ModeloOpal/SM_Master/GR2A AIN (CH00-15) eHS ==
  OP4510_2A_Ch00-07_AIN : rtlab/OpInput  identifier_use=[]  identifier_hide=OP4510_2A_Ch00-07_AIN  nb_parents_identifier=0  passthrough=off  init_value=zeros(1,8)  value_type=double  create_alias=on
      settings: SourceProductName=RT-LAB
  OP4510_2A_Ch08-15_AIN : rtlab/OpInput  identifier_use=[]  identifier_hide=OP4510_2A_Ch08-15_AIN  nb_parents_identifier=0  passthrough=off  init_value=zeros(1,8)  value_type=double  create_alias=on
      settings: SourceProductName=RT-LAB
  Ain1 : Outport
  Ain2 : Outport  Port=2
  wires:
  OP4510_2A_Ch08-15_AIN/1 -> Ain2/1  "AIN CH08-15"
  OP4510_2A_Ch00-07_AIN/1 -> Ain1/1  "AIN CH00-07"

== system ModeloOpal/SM_Master/GenRamp ==
  In1 : Inport
  In2 : Inport  Port=2
  In3 : Inport  Port=3
  Constant3 : Constant  Value=0.8
  Demux5 : Demux  Outputs=3
  Gen Rampa : Subsystem
  OP4510_2B_Ch08-15_AOUT : rtlab/OpOutput  identifier_use=[]  identifier_hide=OP4510_2B_Ch08-15_AOUT  nb_parents_identifier=0
      settings: SourceProductName=RT-LAB
  Product3 : Product  RndMeth=Zero
  Three-phase Sine Wave : Sin  TimeSource=Use external signal  Phase=[0 -2*pi/3 2*pi/3]
  Out1 : Outport
  Out2 : Outport  Port=2
  Out3 : Outport  Port=3
  tag scope: wt=global
  wires:
  Demux5/1 -> Out1/1
  Product3/1 -> Demux5/1
  Demux5/2 -> Out2/1
  Three-phase Sine Wave/1 -> Product3/1
  Constant3/1 -> Product3/2  "<mod_index>"
  Demux5/3 -> Out3/1
  Gen Rampa/1("wt ") -> OP4510_2B_Ch08-15_AOUT/1, [wt], Three-phase Sine Wave/1
  In3/1 -> Gen Rampa/3(En)
  In2/1 -> Gen Rampa/2(Frec)
  In1/1 -> Gen Rampa/1(Fase)

== system ModeloOpal/SM_Master/Id_M ==
  Error : Inport
  En : Inport  Port=2
  Constant2 : Constant  Value=0
  FF Int : DiscreteIntegrator  ExternalReset=level  InitialConditionSource=external  InitialCondition=4  SampleTime=Ts  ICPrevOutput=DiscIntNeverNeededParam  ICPrevScaledInput=DiscIntNeverNeededParam
  Logical Operator : Logic  Operator=NOT  AllPortsSameDT=off  OutDataTypeStr=boolean
  Subsystem : Subsystem
  Subsystem1 : Subsystem
  Sum3 : Sum  OutDataTypeStr=Inherit: Same as first input
  PI : Outport
  wires:
  Subsystem/1(X*Y) -> Sum3/1
  Error/1 -> Subsystem1/1(X), Subsystem/2(Y)
  [Ki_IM] -> Subsystem1/2(Y)
  [Kp_IM] -> Subsystem/1(X)
  Sum3/1 -> PI/1
  En/1 -> Logical Operator/1, Subsystem1/3(En), Subsystem/3(En)
  Logical Operator/1 -> FF Int/2
  Constant2/1 -> FF Int/3
  Subsystem1/1(X*Y) -> FF Int/1
  FF Int/1 -> Sum3/2

== system ModeloOpal/SM_Master/Iq_M ==
  Error : Inport
  En : Inport  Port=2
  Constant2 : Constant  Value=0
  FF Int : DiscreteIntegrator  ExternalReset=level  InitialConditionSource=external  InitialCondition=4  SampleTime=Ts  ICPrevOutput=DiscIntNeverNeededParam  ICPrevScaledInput=DiscIntNeverNeededParam
  Logical Operator : Logic  Operator=NOT  AllPortsSameDT=off  OutDataTypeStr=boolean
  Subsystem : Subsystem
  Subsystem1 : Subsystem
  Sum3 : Sum  OutDataTypeStr=Inherit: Same as first input
  PI : Outport
  wires:
  Subsystem/1(X*Y) -> Sum3/1
  Error/1 -> Subsystem1/1(X), Subsystem/2(Y)
  [Ki_IM] -> Subsystem1/2(Y)
  [Kp_IM] -> Subsystem/1(X)
  Sum3/1 -> PI/1
  En/1 -> Logical Operator/1, Subsystem1/3(En), Subsystem/3(En)
  Logical Operator/1 -> FF Int/2
  Constant2/1 -> FF Int/3
  Subsystem1/1(X*Y) -> FF Int/1
  FF Int/1 -> Sum3/2

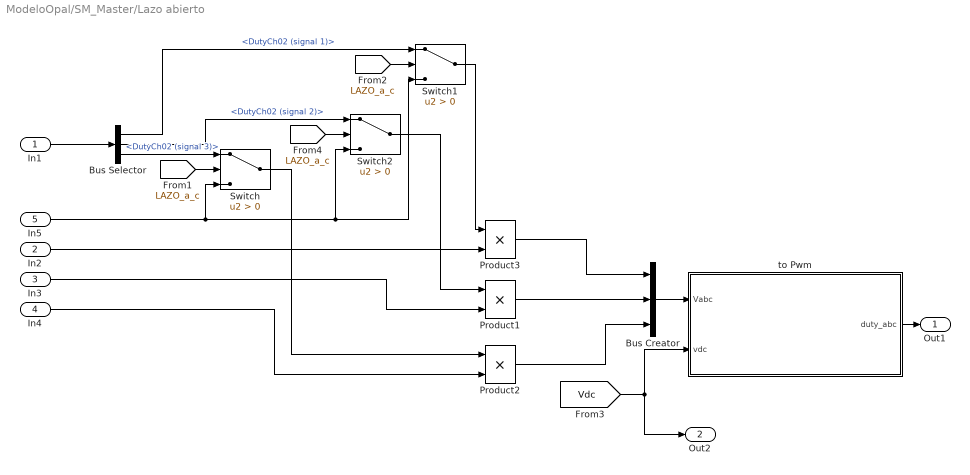
== system ModeloOpal/SM_Master/Lazo abierto  ==
  In1 : Inport
  In2 : Inport  Port=2
  In3 : Inport  Port=3
  In4 : Inport  Port=4
  In5 : Inport  Port=5
  Bus Creator : BusCreator  Inputs=3
  Bus Selector : BusSelector  OutputSignals=DutyCh02 (signal 1),DutyCh02 (signal 2),DutyCh02 (signal 3)
  Product1 : Product  RndMeth=Zero
  Product2 : Product  RndMeth=Zero
  Product3 : Product  RndMeth=Zero
  Switch : Switch  Criteria=u2 > Threshold
  Switch1 : Switch  Criteria=u2 > Threshold
  Switch2 : Switch  Criteria=u2 > Threshold
  to Pwm : Subsystem
      mask Display:
      | disp('Modulation');
      | port_label('input', 1, 'Vpwm');
      | port_label('input', 2, 'Vdc');
      | port_label('output', 1, 'duty');
  Out1 : Outport
  Out2 : Outport  Port=2
  wires:
  In3/1 -> Product1/2
  In4/1 -> Product2/2
  In2/1 -> Product3/2
  [Vdc] -> Out2/1, to Pwm/2(vdc)
  Product3/1 -> Bus Creator/1
  Product1/1 -> Bus Creator/2
  Product2/1 -> Bus Creator/3
  to Pwm/1(duty_abc) -> Out1/1
  Bus Creator/1 -> to Pwm/1(Vabc)
  In1/1 -> Bus Selector/1
  [LAZO_a_c] -> Switch/2
  Bus Selector/3 -> Switch/1  "<DutyCh02 (signal 3)>"
  In5/1 -> Switch1/3, Switch2/3, Switch/3
  [LAZO_a_c] -> Switch1/2
  Switch/1 -> Product2/1
  [LAZO_a_c] -> Switch2/2
  Switch2/1 -> Product1/1
  Bus Selector/2 -> Switch2/1  "<DutyCh02 (signal 2)>"
  Bus Selector/1 -> Switch1/1  "<DutyCh02 (signal 1)>"
  Switch1/1 -> Product3/1

== system ModeloOpal/SM_Master/Parametros de control ==
  Constant : Constant  Value=0.0655
  Constant1 : Constant  Value=22.739
  Constant2 : Constant  Value=20
  Constant3 : Constant  Value=50
  tag scope: Ki_IM=global, Ki_VM=global, Kp_IM=global, Kp_VM=global
  wires:
  Constant3/1 -> [Ki_IM]
  Constant1/1 -> [Ki_VM]
  Constant2/1 -> [Kp_IM]
  Constant/1 -> [Kp_VM]

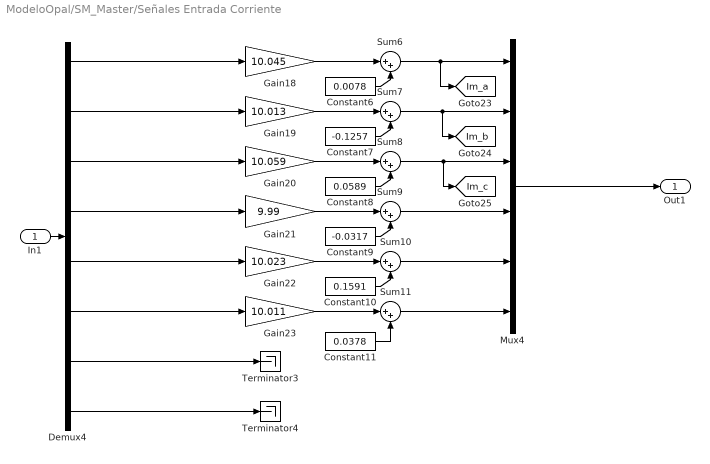
== system ModeloOpal/SM_Master/Señales Entrada Corriente ==
  In1 : Inport
  Constant10 : Constant  Value=0.1591
  Constant11 : Constant  Value=0.0378
  Constant6 : Constant  Value=0.0078
  Constant7 : Constant  Value=-0.1257
  Constant8 : Constant  Value=0.0589
  Constant9 : Constant  Value=-0.0317
  Demux4 : Demux  Outputs=8
  Gain18 : Gain  Gain=10.045
  Gain19 : Gain  Gain=10.013
  Gain20 : Gain  Gain=10.059
  Gain21 : Gain  Gain=9.99
  Gain22 : Gain  Gain=10.023
  Gain23 : Gain  Gain=10.011
  Mux4 : Mux  Inputs=6
  Sum{6..11} (6 alike) : Sum  Inputs=|++
  Terminator3 : Terminator
  Terminator4 : Terminator
  Out1 : Outport
  tag scope: Im_a=global, Im_b=global, Im_c=global
  wires:
  Constant11/1 -> Sum11/2
  Constant7/1 -> Sum7/2
  Sum10/1 -> Mux4/5
  Sum6/1 -> [Im_a], Mux4/1
  Constant10/1 -> Sum10/2
  Gain22/1 -> Sum10/1
  Gain20/1 -> Sum8/1
  Gain21/1 -> Sum9/1
  Sum11/1 -> Mux4/6
  Sum8/1 -> [Im_c], Mux4/3
  Sum7/1 -> [Im_b], Mux4/2
  Constant6/1 -> Sum6/2
  Constant8/1 -> Sum8/2
  Demux4/2 -> Gain19/1
  Constant9/1 -> Sum9/2
  Gain18/1 -> Sum6/1
  Gain19/1 -> Sum7/1
  Sum9/1 -> Mux4/4
  Gain23/1 -> Sum11/1
  Demux4/5 -> Gain22/1
  Demux4/3 -> Gain20/1
  Demux4/4 -> Gain21/1
  Demux4/6 -> Gain23/1
  Demux4/8 -> Terminator4/1
  Demux4/7 -> Terminator3/1
  In1/1 -> Demux4/1
  Mux4/1 -> Out1/1
  Demux4/1 -> Gain18/1

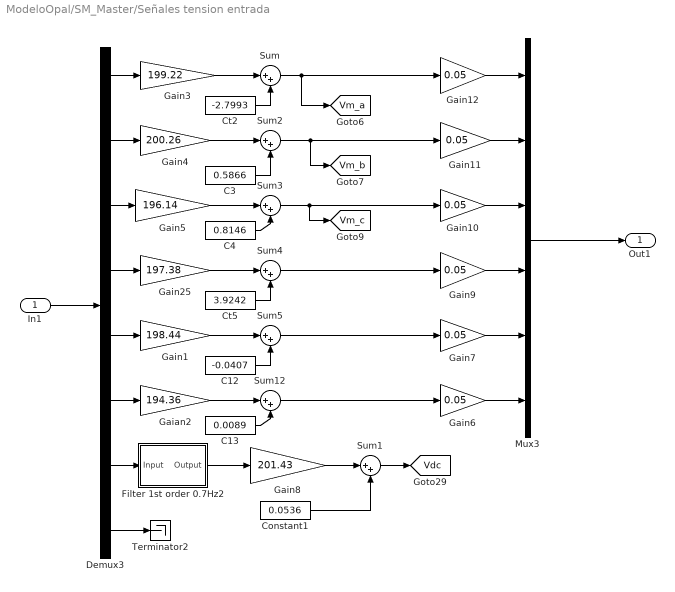
== system ModeloOpal/SM_Master/Señales tension entrada ==
  In1 : Inport
  C12 : Constant  Value=-0.0407
  C13 : Constant  Value=0.0089
  C3 : Constant  Value=0.5866
  C4 : Constant  Value=0.8146
  Constant1 : Constant  Value=0.0536
  Ct2 : Constant  Value=-2.7993
  Ct5 : Constant  Value=3.9242
  Demux3 : Demux  Outputs=8
  Filter 1st order 0.7Hz2 : Subsystem  Tag=FilterWizardSubSystem
      settings: ErrorFcn=dspFilterRealizedInBasicElemsAlgLoopErrFcnCallback
  Gaian2 : Gain  Gain=194.36
  Gain1 : Gain  Gain=198.44
  Gain{6..7,9..12} (6 alike) : Gain  Gain=0.05
  Gain25 : Gain  Gain=197.38
  Gain3 : Gain  Gain=199.22
  Gain4 : Gain  Gain=200.26
  Gain5 : Gain  Gain=196.14
  Gain8 : Gain  Gain=201.43
  Mux3 : Mux  Inputs=6
  Sum{,1..5,12} (7 alike) : Sum  Inputs=|++
  Terminator2 : Terminator
  Out1 : Outport
  tag scope: Vdc=global, Vm_a=global, Vm_b=global, Vm_c=global
  wires:
  Gaian2/1 -> Sum12/1
  Sum12/1 -> Gain6/1
  C12/1 -> Sum5/2
  Sum5/1 -> Gain7/1
  Constant1/1 -> Sum1/2
  Sum1/1 -> [Vdc]
  Gain25/1 -> Sum4/1
  Gain1/1 -> Sum5/1
  C13/1 -> Sum12/2
  Sum/1 -> [Vm_a], Gain12/1
  Sum2/1 -> [Vm_b], Gain11/1
  Sum3/1 -> Gain10/1, [Vm_c]
  Gain5/1 -> Sum3/1
  Ct5/1 -> Sum4/2
  Gain8/1 -> Sum1/1
  Ct2/1 -> Sum/2
  Sum4/1 -> Gain9/1
  C3/1 -> Sum2/2
  C4/1 -> Sum3/2
  Gain4/1 -> Sum2/1
  Demux3/4 -> Gain25/1
  Demux3/3 -> Gain5/1
  Demux3/6 -> Gaian2/1
  Gain3/1 -> Sum/1
  Demux3/1 -> Gain3/1
  Demux3/5 -> Gain1/1
  Demux3/2 -> Gain4/1
  Demux3/8 -> Terminator2/1
  Mux3/1 -> Out1/1
  Filter 1st order 0.7Hz2/1(Output) -> Gain8/1
  In1/1 -> Demux3/1
  Demux3/7 -> Filter 1st order 0.7Hz2/1(Input)
  Gain6/1 -> Mux3/6
  Gain7/1 -> Mux3/5
  Gain9/1 -> Mux3/4
  Gain10/1 -> Mux3/3
  Gain11/1 -> Mux3/2
  Gain12/1 -> Mux3/1

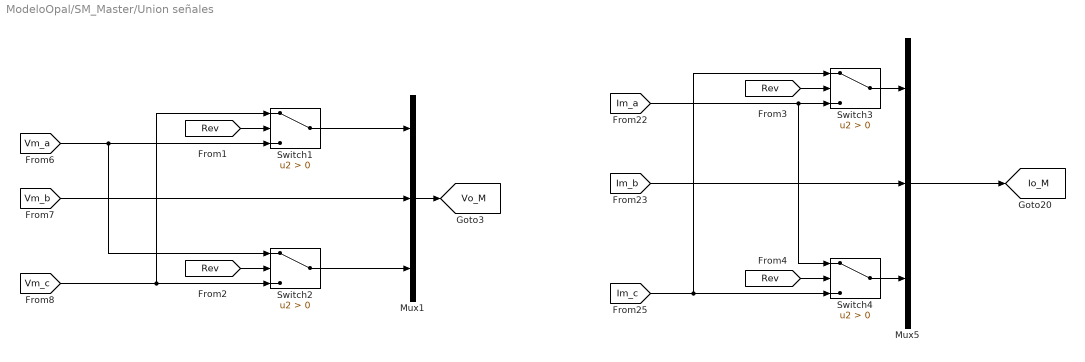
== system ModeloOpal/SM_Master/Union señales  ==
  Mux1 : Mux  Inputs=3
  Mux5 : Mux  Inputs=3
  Switch{1..4} (4 alike) : Switch  Criteria=u2 > Threshold
  tag scope: Io_M=global, Vo_M=global
  wires:
  Mux5/1 -> [Io_M]
  Mux1/1 -> [Vo_M]
  [Vm_b] -> Mux1/2
  [Rev] -> Switch1/2
  [Vm_a] -> Switch2/1, Switch1/3
  [Rev] -> Switch2/2
  [Vm_c] -> Switch1/1, Switch2/3
  Switch1/1 -> Mux1/1
  Switch2/1 -> Mux1/3
  [Im_b] -> Mux5/2
  [Rev] -> Switch3/2
  Switch3/1 -> Mux5/1
  [Im_a] -> Switch4/1, Switch3/3
  [Rev] -> Switch4/2
  Switch4/1 -> Mux5/3
  [Im_c] -> Switch3/1, Switch4/3

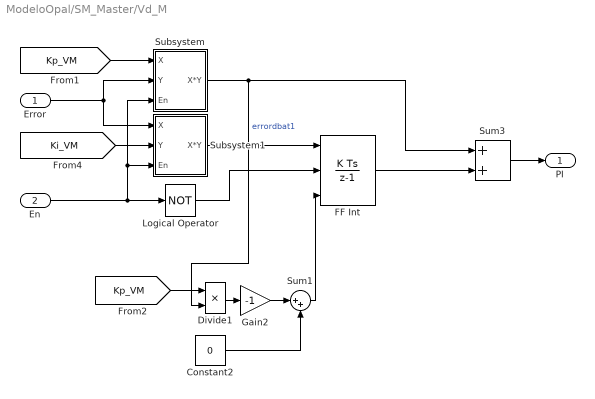
== system ModeloOpal/SM_Master/Vd_M ==
  Error : Inport
  En : Inport  Port=2
  Constant2 : Constant  Value=0
  Divide1 : Product  Inputs=**  OutDataTypeStr=Inherit: Same as first input
  FF Int : DiscreteIntegrator  ExternalReset=level  InitialConditionSource=external  InitialCondition=4  SampleTime=Ts  ICPrevOutput=DiscIntNeverNeededParam  ICPrevScaledInput=DiscIntNeverNeededParam
  Gain2 : Gain  Gain=-1
  Logical Operator : Logic  Operator=NOT  AllPortsSameDT=off  OutDataTypeStr=boolean
  Subsystem : Subsystem
  Subsystem1 : Subsystem
  Sum1 : Sum  Inputs=|++
  Sum3 : Sum  OutDataTypeStr=Inherit: Same as first input
  PI : Outport
  wires:
  Error/1 -> Subsystem1/1(X), Subsystem/2(Y)
  [Ki_VM] -> Subsystem1/2(Y)
  [Kp_VM] -> Subsystem/1(X)
  Sum3/1 -> PI/1
  En/1 -> Logical Operator/1, Subsystem1/3(En), Subsystem/3(En)
  Logical Operator/1 -> FF Int/2
  Gain2/1 -> Sum1/1
  [Kp_VM] -> Divide1/1
  Divide1/1 -> Gain2/1
  Subsystem/1(X*Y) -> Divide1/2, Sum3/1  "errordbat1"
  Sum1/1 -> FF Int/3
  Constant2/1 -> Sum1/2
  Subsystem1/1(X*Y) -> FF Int/1
  FF Int/1 -> Sum3/2

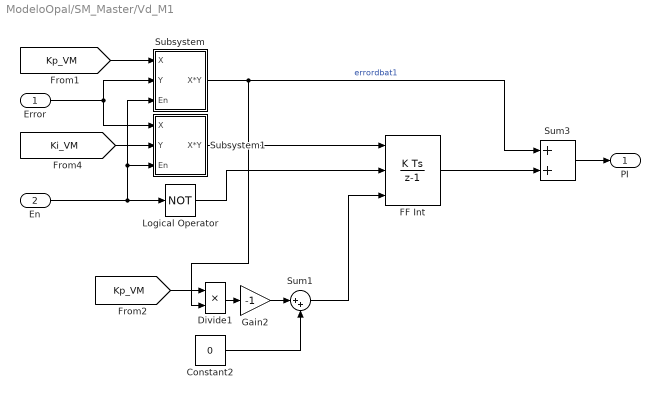
== system ModeloOpal/SM_Master/Vd_M1 ==
  Error : Inport
  En : Inport  Port=2
  Constant2 : Constant  Value=0
  Divide1 : Product  Inputs=**  OutDataTypeStr=Inherit: Same as first input
  FF Int : DiscreteIntegrator  ExternalReset=level  InitialConditionSource=external  InitialCondition=4  SampleTime=Ts  ICPrevOutput=DiscIntNeverNeededParam  ICPrevScaledInput=DiscIntNeverNeededParam
  Gain2 : Gain  Gain=-1
  Logical Operator : Logic  Operator=NOT  AllPortsSameDT=off  OutDataTypeStr=boolean
  Subsystem : Subsystem
  Subsystem1 : Subsystem
  Sum1 : Sum  Inputs=|++
  Sum3 : Sum  OutDataTypeStr=Inherit: Same as first input
  PI : Outport
  wires:
  Error/1 -> Subsystem1/1(X), Subsystem/2(Y)
  [Ki_VM] -> Subsystem1/2(Y)
  [Kp_VM] -> Subsystem/1(X)
  Sum3/1 -> PI/1
  En/1 -> Logical Operator/1, Subsystem1/3(En), Subsystem/3(En)
  Logical Operator/1 -> FF Int/2
  Gain2/1 -> Sum1/1
  [Kp_VM] -> Divide1/1
  Divide1/1 -> Gain2/1
  Subsystem/1(X*Y) -> Divide1/2, Sum3/1  "errordbat1"
  Sum1/1 -> FF Int/3
  Constant2/1 -> Sum1/2
  Subsystem1/1(X*Y) -> FF Int/1
  FF Int/1 -> Sum3/2

== system ModeloOpal/SM_Master/abc//dq_VM ==
  abc : Inport
  wt : Inport  Port=2
  Subsystem2 : Subsystem
  abc/alfabeta2 : Subsystem  mask{k=2/3}
  d : Outport
  Q : Outport  Port=2
  wires:
  abc/alfabeta2/1(alfa) -> Subsystem2/1(alfa)
  abc/alfabeta2/2(Beta) -> Subsystem2/2(beta)
  wt/1 -> Subsystem2/3(wt)
  Subsystem2/2(Q) -> Q/1
  abc/1 -> abc/alfabeta2/1(abc)
  Subsystem2/1(d) -> d/1

== system ModeloOpal/SM_Master/abc//dq_VM1 ==
  abc : Inport
  wt : Inport  Port=2
  Subsystem2 : Subsystem
  abc/alfabeta2 : Subsystem  mask{k=2/3}
  d : Outport
  Q : Outport  Port=2
  wires:
  Subsystem2/1(d) -> d/1
  abc/1 -> abc/alfabeta2/1(abc)
  Subsystem2/2(Q) -> Q/1
  wt/1 -> Subsystem2/3(wt)
  abc/alfabeta2/2(Beta) -> Subsystem2/2(beta)
  abc/alfabeta2/1(alfa) -> Subsystem2/1(alfa)

== system ModeloOpal/SM_Master/dq//abc ==
  d : Inport
  q : Inport  Port=2
  wt : Inport  Port=3
  Subsystem1 : Subsystem  mask{k=1}
  dq/alfabeta1 : Subsystem
  a : Outport
  b : Outport  Port=2
  c : Outport  Port=3
  wires:
  dq/alfabeta1/1(alfa) -> Subsystem1/1(alfa)
  dq/alfabeta1/2(beta) -> Subsystem1/2(beta)
  wt/1 -> dq/alfabeta1/3(wt)
  d/1 -> dq/alfabeta1/1(d)
  Subsystem1/1(a) -> a/1
  Subsystem1/3(c) -> c/1
  Subsystem1/2(b) -> b/1
  q/1 -> dq/alfabeta1/2(q)

== system ModeloOpal/SM_Master/eHS AO16ch_AI16ch ==
  AOUT : Inport
  AOUT1 : Inport  Port=2
  Demux : Demux  Outputs=6
  Demux1 : Demux  Outputs=6
  OP4510_2B_Ch00-07_AOUT : rtlab/OpOutput  identifier_use=[]  identifier_hide=OP4510_2B_Ch00-07_AOUT  nb_parents_identifier=0
      settings: SourceProductName=RT-LAB
  OP4510_2B_Ch00-07_AOUT1 : rtlab/OpOutput  identifier_use=[]  identifier_hide=OP4510_2B_Ch00-07_AOUT1  nb_parents_identifier=0
      settings: SourceProductName=RT-LAB
  OP4510_2B_Ch00-07_AOUT2 : rtlab/OpOutput  identifier_use=[]  identifier_hide=OP4510_2B_Ch00-07_AOUT2  nb_parents_identifier=0
      settings: SourceProductName=RT-LAB
  OP4510_2B_Ch00-07_AOUT3 : rtlab/OpOutput  identifier_use=[]  identifier_hide=OP4510_2B_Ch00-07_AOUT3  nb_parents_identifier=0
      settings: SourceProductName=RT-LAB
  OP4510_2B_Ch00-07_AOUT4 : rtlab/OpOutput  identifier_use=[]  identifier_hide=OP4510_2B_Ch00-07_AOUT4  nb_parents_identifier=0
      settings: SourceProductName=RT-LAB
  OP4510_2B_Ch00-07_AOUT5 : rtlab/OpOutput  identifier_use=[]  identifier_hide=OP4510_2B_Ch00-07_AOUT5  nb_parents_identifier=0
      settings: SourceProductName=RT-LAB
  wires:
  AOUT/1 -> Demux/1
  AOUT1/1 -> Demux1/1
  Demux/2 -> OP4510_2B_Ch00-07_AOUT1/1
  Demux/3 -> OP4510_2B_Ch00-07_AOUT2/1
  Demux/1 -> OP4510_2B_Ch00-07_AOUT/1
  Demux1/2 -> OP4510_2B_Ch00-07_AOUT4/1
  Demux1/1 -> OP4510_2B_Ch00-07_AOUT3/1
  Demux1/3 -> OP4510_2B_Ch00-07_AOUT5/1

== system ModeloOpal/SM_Master/to pwm_M ==
  In1 : Inport
  In2 : Inport  Port=2
  Bus Creator2 : BusCreator  Inputs=3
  Demux1 : Demux  Outputs=3
  Salida PWM : Subsystem
  to Pwm1 : Subsystem
      mask Display:
      | disp('Modulation');
      | port_label('input', 1, 'Vpwm');
      | port_label('input', 2, 'Vdc');
      | port_label('output', 1, 'duty');
  wires:
  In1/1 -> to Pwm1/1(Vabc)
  Demux1/3 -> Bus Creator2/3
  Demux1/1 -> Bus Creator2/1
  Bus Creator2/1 -> Salida PWM/2("ciclo util ")
  In2/1 -> to Pwm1/2(vdc)
  Demux1/2 -> Bus Creator2/2
  [Frecuencia] -> Salida PWM/1(Frecuencia)
  to Pwm1/1(duty_abc) -> Demux1/1

== system ModeloOpal/SM_Master/Calculadora Potencia/Clarke Transformation1 ==
  v-abc : Inport
  Clarke to Beta : Fcn  Expr=0*u[1]+sqrt(1/2)*u[2]-sqrt(1/2)*u[3]
  Clarke to alpha : Fcn  Expr=sqrt(2/3)*u[1]-sqrt(1/6)*u[2]-sqrt(1/6)*u[3]
  v-alpha : Outport
  v-beta : Outport  Port=2
  wires:
  Clarke to Beta/1 -> v-beta/1
  Clarke to alpha/1 -> v-alpha/1
  v-abc/1 -> Clarke to Beta/1, Clarke to alpha/1

== system ModeloOpal/SM_Master/Calculadora Potencia/Clarke Transformation2 ==
  v-abc : Inport
  Clarke to Beta : Fcn  Expr=0*u[1]+sqrt(1/2)*u[2]-sqrt(1/2)*u[3]
  Clarke to alpha : Fcn  Expr=sqrt(2/3)*u[1]-sqrt(1/6)*u[2]-sqrt(1/6)*u[3]
  v-alpha : Outport
  v-beta : Outport  Port=2
  wires:
  v-abc/1 -> Clarke to alpha/1, Clarke to Beta/1
  Clarke to alpha/1 -> v-alpha/1
  Clarke to Beta/1 -> v-beta/1

== system ModeloOpal/SM_Master/Calculadora Potencia/Filter 1st order 0.7Hz1 ==
  Input : Inport
  Delay11 : Delay  DelayLength=1  InitialCondition=0  InputProcessing=Inherited
  SumA21 : Sum  Inputs=|+-  RndMeth=Nearest  SaturateOnIntegerOverflow=on  OutDataTypeStr=Inherit: Same as first input
  SumB21 : Sum  Inputs=|++  RndMeth=Nearest  SaturateOnIntegerOverflow=on  OutDataTypeStr=Inherit: Same as first input
  a(2)(1) : Gain  Gain=-0.99956027372226808  ParamDataTypeStr=float('double')  RndMeth=Nearest  SaturateOnIntegerOverflow=on  OutDataTypeStr=Inherit: Same as input
  s(1) : Gain  Gain=0.00021986313886602718  ParamDataTypeStr=float('double')  RndMeth=Nearest  SaturateOnIntegerOverflow=on  OutDataTypeStr=Inherit: Same as input
  Output : Outport
  wires:
  Delay11/1 -> SumB21/2, a(2)(1)/1
  a(2)(1)/1 -> SumA21/2
  SumB21/1 -> Output/1
  SumA21/1 -> Delay11/1, SumB21/1
  s(1)/1 -> SumA21/1
  Input/1 -> s(1)/1

== system ModeloOpal/SM_Master/Calculadora Potencia/Filter 1st order 0.7Hz2 ==
  Input : Inport
  Delay11 : Delay  DelayLength=1  InitialCondition=0  InputProcessing=Inherited
  SumA21 : Sum  Inputs=|+-  RndMeth=Nearest  SaturateOnIntegerOverflow=on  OutDataTypeStr=Inherit: Same as first input
  SumB21 : Sum  Inputs=|++  RndMeth=Nearest  SaturateOnIntegerOverflow=on  OutDataTypeStr=Inherit: Same as first input
  a(2)(1) : Gain  Gain=-0.99956027372226808  ParamDataTypeStr=float('double')  RndMeth=Nearest  SaturateOnIntegerOverflow=on  OutDataTypeStr=Inherit: Same as input
  s(1) : Gain  Gain=0.00021986313886602718  ParamDataTypeStr=float('double')  RndMeth=Nearest  SaturateOnIntegerOverflow=on  OutDataTypeStr=Inherit: Same as input
  Output : Outport
  wires:
  Input/1 -> s(1)/1
  s(1)/1 -> SumA21/1
  SumA21/1 -> SumB21/1, Delay11/1
  SumB21/1 -> Output/1
  a(2)(1)/1 -> SumA21/2
  Delay11/1 -> a(2)(1)/1, SumB21/2

== system ModeloOpal/SM_Master/GenRamp/Gen Rampa ==
  Fase : Inport
  Frec : Inport  Port=2
  En : Inport  Port=3
  Add1 : Sum
  Compare To Constant1 : simulink/Logic and Bit Operations/Compare To Constant  relop=>=  const=2*pi  OutDataTypeStr=boolean
  Gain : Gain  Gain=2*pi
  Gain6 : Gain  Gain=pi/180
  Integrator : Integrator  ExternalReset=rising
  Product : Product
  Unit Delay2 : UnitDelay  SampleTime=Ts
  "wt " : Outport
  wires:
  Unit Delay2/1 -> Integrator/2
  Add1/1 -> "wt "/1
  En/1 -> Product/2
  Gain6/1 -> Add1/1
  Compare To Constant1/1 -> Unit Delay2/1
  Fase/1 -> Gain6/1
  Gain/1 -> Product/1
  Product/1 -> Integrator/1
  Integrator/1 -> Add1/2, Compare To Constant1/1
  Frec/1 -> Gain/1

== system ModeloOpal/SM_Master/Id_M/Subsystem ==
  X : Inport
  Y : Inport  Port=2
  En : Inport  Port=3
  Divide2 : Product  Inputs=**  OutDataTypeStr=Inherit: Same as first input
  Divide5 : Product  Inputs=**  OutDataTypeStr=Inherit: Same as first input
  X*Y : Outport
  wires:
  X/1 -> Divide2/1
  En/1 -> Divide5/2
  Divide2/1 -> Divide5/1
  Divide5/1 -> X*Y/1
  Y/1 -> Divide2/2

== system ModeloOpal/SM_Master/Id_M/Subsystem1 ==
  X : Inport
  Y : Inport  Port=2
  En : Inport  Port=3
  Divide2 : Product  Inputs=**  OutDataTypeStr=Inherit: Same as first input
  Divide5 : Product  Inputs=**  OutDataTypeStr=Inherit: Same as first input
  X*Y : Outport
  wires:
  X/1 -> Divide2/1
  En/1 -> Divide5/2
  Divide2/1 -> Divide5/1
  Divide5/1 -> X*Y/1
  Y/1 -> Divide2/2

== system ModeloOpal/SM_Master/Iq_M/Subsystem ==
  X : Inport
  Y : Inport  Port=2
  En : Inport  Port=3
  Divide2 : Product  Inputs=**  OutDataTypeStr=Inherit: Same as first input
  Divide5 : Product  Inputs=**  OutDataTypeStr=Inherit: Same as first input
  X*Y : Outport
  wires:
  X/1 -> Divide2/1
  En/1 -> Divide5/2
  Divide2/1 -> Divide5/1
  Divide5/1 -> X*Y/1
  Y/1 -> Divide2/2

== system ModeloOpal/SM_Master/Iq_M/Subsystem1 ==
  X : Inport
  Y : Inport  Port=2
  En : Inport  Port=3
  Divide2 : Product  Inputs=**  OutDataTypeStr=Inherit: Same as first input
  Divide5 : Product  Inputs=**  OutDataTypeStr=Inherit: Same as first input
  X*Y : Outport
  wires:
  X/1 -> Divide2/1
  En/1 -> Divide5/2
  Divide2/1 -> Divide5/1
  Divide5/1 -> X*Y/1
  Y/1 -> Divide2/2

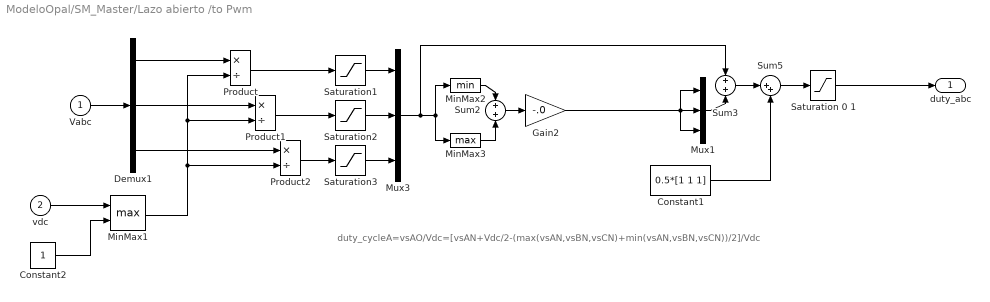
== system ModeloOpal/SM_Master/Lazo abierto /to Pwm ==
  note: duty_cycleA=vsAO/Vdc=[vsAN+Vdc/2-(max(vsAN,vsBN,vsCN)+min(vsAN,vsBN,vsCN))/2]/Vdc
  Vabc : Inport
  vdc : Inport  Port=2
  Constant1 : Constant  Value=0.5*[1 1 1]
  Constant2 : Constant
  Demux1 : Demux  Outputs=3
  Gain2 : Gain  Gain=-.0  SaturateOnIntegerOverflow=on  OutDataTypeStr=Inherit: Same as input  ParamDataTypeStr=Inherit: Same as input
  MinMax1 : MinMax  Function=max  Inputs=2  SaturateOnIntegerOverflow=on  InputSameDT=on
  MinMax2 : MinMax  SaturateOnIntegerOverflow=on  InputSameDT=on
  MinMax3 : MinMax  Function=max  SaturateOnIntegerOverflow=on  InputSameDT=on
  Mux1 : Mux  Inputs=3
  Mux3 : Mux  Inputs=3
  Product : Product  Inputs=*/  SaturateOnIntegerOverflow=on  OutDataTypeStr=Inherit: Same as first input
  Product1 : Product  Inputs=*/  SaturateOnIntegerOverflow=on  OutDataTypeStr=Inherit: Same as first input
  Product2 : Product  Inputs=*/  SaturateOnIntegerOverflow=on  OutDataTypeStr=Inherit: Same as first input
  Saturation 0 1 : Saturate  UpperLimit=0.98  LowerLimit=0.02
  Saturation1 : Saturate  UpperLimit=1/sqrt(3)  LowerLimit=-1/sqrt(3)
  Saturation2 : Saturate  UpperLimit=1/sqrt(3)  LowerLimit=-1/sqrt(3)
  Saturation3 : Saturate  UpperLimit=1/sqrt(3)  LowerLimit=-1/sqrt(3)
  Sum2 : Sum  SaturateOnIntegerOverflow=on  InputSameDT=on  OutDataTypeStr=Inherit: Same as first input
  Sum3 : Sum  SaturateOnIntegerOverflow=on  InputSameDT=on  OutDataTypeStr=Inherit: Same as first input
  Sum5 : Sum  Inputs=|++  SaturateOnIntegerOverflow=on  InputSameDT=on  OutDataTypeStr=Inherit: Same as first input
  duty_abc : Outport
  wires:
  Sum5/1 -> Saturation 0 1/1
  Mux3/1 -> MinMax3/1, MinMax2/1, Sum3/1
  MinMax3/1 -> Sum2/2
  MinMax2/1 -> Sum2/1
  Sum2/1 -> Gain2/1
  Gain2/1 -> Mux1/2, Mux1/3, Mux1/1
  Sum3/1 -> Sum5/1
  Constant1/1 -> Sum5/2
  Demux1/3 -> Product2/1
  Demux1/1 -> Product/1
  Saturation1/1 -> Mux3/1
  Saturation2/1 -> Mux3/2
  Saturation3/1 -> Mux3/3
  Product/1 -> Saturation1/1
  Product1/1 -> Saturation2/1
  Demux1/2 -> Product1/1
  Product2/1 -> Saturation3/1
  Saturation 0 1/1 -> duty_abc/1
  Mux1/1 -> Sum3/2
  vdc/1 -> MinMax1/1
  MinMax1/1 -> Product2/2, Product1/2, Product/2
  Constant2/1 -> MinMax1/2
  Vabc/1 -> Demux1/1

== system ModeloOpal/SM_Master/Señales tension entrada/Filter 1st order 0.7Hz2 ==
  Input : Inport
  Delay11 : Delay  DelayLength=1  InitialCondition=0  InputProcessing=Inherited
  SumA21 : Sum  Inputs=|+-  RndMeth=Nearest  SaturateOnIntegerOverflow=on  OutDataTypeStr=Inherit: Same as first input
  SumB21 : Sum  Inputs=|++  RndMeth=Nearest  SaturateOnIntegerOverflow=on  OutDataTypeStr=Inherit: Same as first input
  a(2)(1) : Gain  Gain=-0.99956027372226808  ParamDataTypeStr=float('double')  RndMeth=Nearest  SaturateOnIntegerOverflow=on  OutDataTypeStr=Inherit: Same as input
  s(1) : Gain  Gain=0.00021986313886602718  ParamDataTypeStr=float('double')  RndMeth=Nearest  SaturateOnIntegerOverflow=on  OutDataTypeStr=Inherit: Same as input
  Output : Outport
  wires:
  Delay11/1 -> SumB21/2, a(2)(1)/1
  a(2)(1)/1 -> SumA21/2
  SumB21/1 -> Output/1
  SumA21/1 -> Delay11/1, SumB21/1
  s(1)/1 -> SumA21/1
  Input/1 -> s(1)/1

== system ModeloOpal/SM_Master/Vd_M/Subsystem ==
  X : Inport
  Y : Inport  Port=2
  En : Inport  Port=3
  Divide2 : Product  Inputs=**  OutDataTypeStr=Inherit: Same as first input
  Divide5 : Product  Inputs=**  OutDataTypeStr=Inherit: Same as first input
  X*Y : Outport
  wires:
  X/1 -> Divide2/1
  En/1 -> Divide5/2
  Divide2/1 -> Divide5/1
  Divide5/1 -> X*Y/1
  Y/1 -> Divide2/2
